simulink library "Transmission_Validation"  (R2017a)
settings: Solver=VariableStepAuto  StartTime=0.0  StopTime=10.0  RelTol=1e-3
undefined symbols (not defined in the file): BrkPdlPos_Data, EngActStdyStTorq_Da, EngSpd_Data, ThrPos_Data, Time_Data, TransEstGear_Data, TrnsOutShftAngVel_D, TrnTrbAngVl_Data
settings Model: Creator=Di Russo  LastModifiedBy=Di Russo

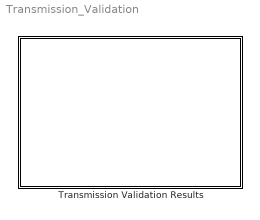
== system Transmission_Validation ==
  Transmission Validation Results : Subsystem
      mask Display: image('Images\Scope.jpg')

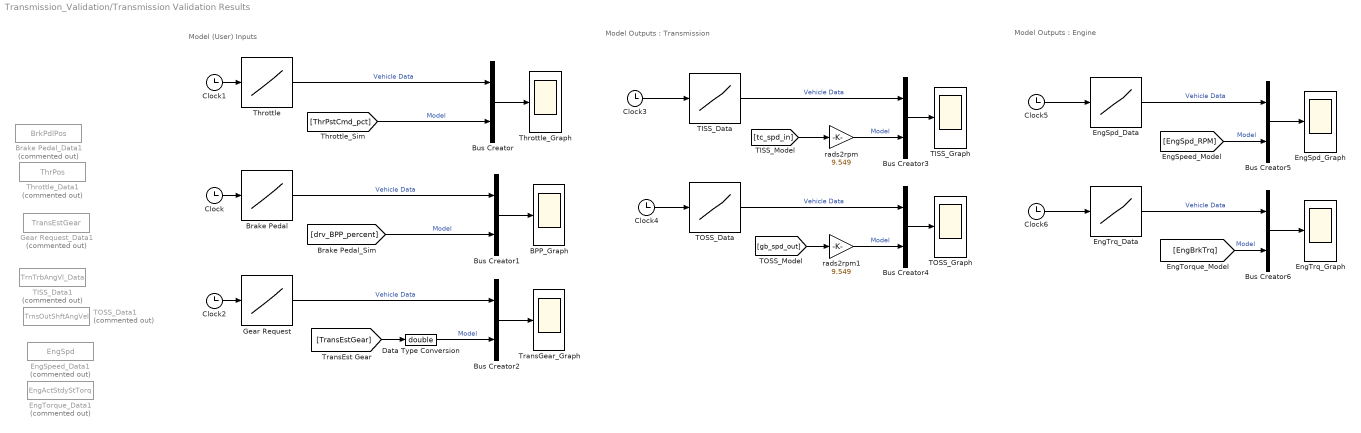
== system Transmission_Validation/Transmission Validation Results ==
  note: Model Outputs : Engine
  note: Model Outputs : Transmission
  note: Model (User) Inputs
  BPP_Graph : Scope
  Brake Pedal : Lookup_n-D  NumberOfTableDimensions=1  BreakpointsForDimension1=Time_Data  Table=BrkPdlPos_Data  InternalRulePriority=Speed  RndMeth=Simplest  InputSameDT=on
  Brake Pedal_Data1 : FromWorkspace  Commented=on  VariableName=BrkPdlPos  OutDataTypeStr=double  SampleTime=0
  Bus Creator{,1..6} (7 alike) : BusCreator  Inputs=2
  Clock{,1..6} (7 alike) : Clock
  Data Type Conversion : DataTypeConversion  OutDataTypeStr=double
  EngSpd_Data : Lookup_n-D  NumberOfTableDimensions=1  BreakpointsForDimension1=Time_Data  Table=EngSpd_Data  InternalRulePriority=Speed  RndMeth=Simplest  InputSameDT=on
  EngSpd_Graph : Scope
  EngSpeed_Data1 : FromWorkspace  Commented=on  VariableName=EngSpd  SampleTime=0
  EngTorque_Data1 : FromWorkspace  Commented=on  VariableName=EngActStdyStTorq  SampleTime=0
  EngTrq_Data : Lookup_n-D  NumberOfTableDimensions=1  BreakpointsForDimension1=Time_Data  Table=EngActStdyStTorq_Da  InternalRulePriority=Speed  RndMeth=Simplest  InputSameDT=on
  EngTrq_Graph : Scope
  Gear Request : Lookup_n-D  NumberOfTableDimensions=1  BreakpointsForDimension1=Time_Data  Table=TransEstGear_Data  InternalRulePriority=Speed  RndMeth=Simplest  InputSameDT=on
  Gear Request_Data1 : FromWorkspace  Commented=on  VariableName=TransEstGear  SampleTime=0
  TISS_Data : Lookup_n-D  NumberOfTableDimensions=1  BreakpointsForDimension1=Time_Data  Table=TrnTrbAngVl_Data  InternalRulePriority=Speed  RndMeth=Simplest  InputSameDT=on
  TISS_Data1 : FromWorkspace  Commented=on  VariableName=TrnTrbAngVl_Data  SampleTime=0
  TISS_Graph : Scope
  TOSS_Data : Lookup_n-D  NumberOfTableDimensions=1  BreakpointsForDimension1=Time_Data  Table=TrnsOutShftAngVel_D  InternalRulePriority=Speed  RndMeth=Simplest  InputSameDT=on
  TOSS_Data1 : FromWorkspace  Commented=on  VariableName=TrnsOutShftAngVel  SampleTime=0
  TOSS_Graph : Scope
  Throttle : Lookup_n-D  NumberOfTableDimensions=1  BreakpointsForDimension1=Time_Data  Table=ThrPos_Data  InternalRulePriority=Speed  RndMeth=Simplest  InputSameDT=on
  Throttle_Data1 : FromWorkspace  Commented=on  VariableName=ThrPos  SampleTime=0
  Throttle_Graph : Scope
  TransGear_Graph : Scope
  rads2rpm : Gain  Gain=9.549
  rads2rpm1 : Gain  Gain=9.549
  wires:
  [ThrPstCmd_pct] -> Bus Creator/2  "Model"
  Bus Creator/1 -> Throttle_Graph/1
  [drv_BPP_percent] -> Bus Creator1/2  "Model"
  Brake Pedal/1 -> Bus Creator1/1  "Vehicle Data"
  Bus Creator1/1 -> BPP_Graph/1
  [TransEstGear] -> Data Type Conversion/1
  Bus Creator2/1 -> TransGear_Graph/1
  [tc_spd_in] -> rads2rpm/1
  Bus Creator3/1 -> TISS_Graph/1
  Bus Creator4/1 -> TOSS_Graph/1
  TOSS_Data/1 -> Bus Creator4/1  "Vehicle Data"
  rads2rpm1/1 -> Bus Creator4/2  "Model"
  [EngSpd_RPM] -> Bus Creator5/2  "Model"
  EngSpd_Data/1 -> Bus Creator5/1  "Vehicle Data"
  Bus Creator5/1 -> EngSpd_Graph/1
  EngTrq_Data/1 -> Bus Creator6/1  "Vehicle Data"
  Bus Creator6/1 -> EngTrq_Graph/1
  [EngBrkTrq] -> Bus Creator6/2  "Model"
  Clock/1 -> Brake Pedal/1
  Throttle/1 -> Bus Creator/1  "Vehicle Data"
  Clock1/1 -> Throttle/1
  Clock2/1 -> Gear Request/1
  Gear Request/1 -> Bus Creator2/1  "Vehicle Data"
  Data Type Conversion/1 -> Bus Creator2/2  "Model"
  Clock3/1 -> TISS_Data/1
  TISS_Data/1 -> Bus Creator3/1  "Vehicle Data"
  Clock4/1 -> TOSS_Data/1
  rads2rpm/1 -> Bus Creator3/2  "Model"
  [gb_spd_out] -> rads2rpm1/1
  Clock5/1 -> EngSpd_Data/1
  Clock6/1 -> EngTrq_Data/1
